simulink model "SistemaP1"  (R2023a)
settings: Solver=VariableStepAuto  StartTime=0.0  StopTime=10  RelTol=1e-3
libraries: slpidlib x1, simulink x1
settings Model: LastModifiedBy=biom3
settings DataIOCC: SaveOutput=off  ReturnWorkspaceOutputs=off  TimeSaveName=t
settings DebuggingCC: AlgebraicLoopMsg=none  ArtificialAlgebraicLoopMsg=none  InheritedTsInSrcMsg=none  MultiTaskCondExecSysMsg=none  TasksWithSamePriorityMsg=none  SigSpecEnsureSampleTimeMsg=none  UnknownTsInhSupMsg=none
settings RTWCC: GPUComputeCapability=5.0

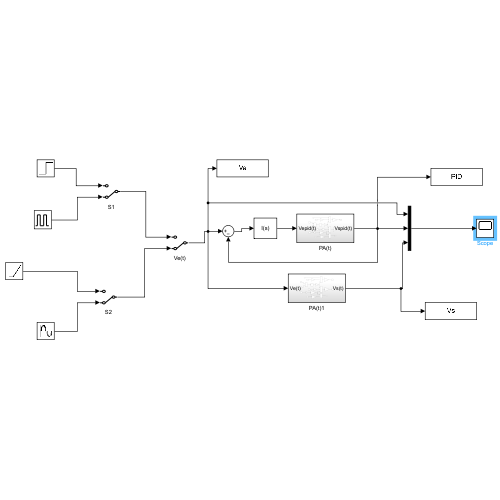
[thumbnail: Simulink's stored preview of the top-level diagram]
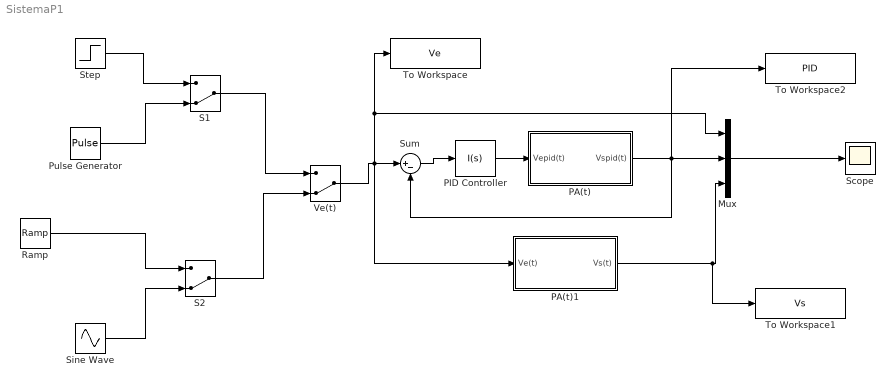
== system SistemaP1 ==
  Mux : Mux  Inputs=3
  PA(t) : Subsystem
  PA(t)1 : Subsystem
  PID Controller : slpidlib/PID Controller  Controller=I  Form=Parallel  TimeDomain=Continuous-time  UseExternalTs=off  SampleTime=-1  IntegratorMethod=Forward Euler  FilterMethod=Forward Euler  ControllerParametersSource=internal  P=1  I=731.453807138668  UseKiTs=off  D=1  N=1  UseFilter=on  TunerSelectOption=Transfer Function Based (PID Tuner App)  InitialConditionSource=internal  InitialConditionForIntegrator=0  InitialConditionForFilter=0  DifferentiatorICPrevScaledInput=0  ExternalReset=none  TrackingMode=off  Kt=1  LimitOutput=off  SatLimitsSource=internal  UpperSaturationLimit=inf  LowerSaturationLimit=-inf  LinearizeAsGain=on  AntiWindupMode=none  Kb=1  LimitIntegrator=off  UpperIntegratorSaturationLimit=inf  LowerIntegratorSaturationLimit=-inf  POutMin=[]  POutMax=[]  IOutMin=[]  IOutMax=[]  DOutMin=[]  DOutMax=[]  NOutMin=[]  NOutMax=[]  SumOutMin=[]  SumOutMax=[]  SaturationOutMin=[]  SaturationOutMax=[]  PParamMin=[]  PParamMax=[]  IParamMin=[]  IParamMax=[]  DParamMin=[]  DParamMax=[]  NParamMin=[]  NParamMax=[]  KbParamMin=[]  KbParamMax=[]  KtParamMin=[]  KtParamMax=[]  KbOutMin=[]  KbOutMax=[]  KtOutMin=[]  KtOutMax=[]  IntegratorOutMin=[]  IntegratorOutMax=[]  FilterOutMin=[]  FilterOutMax=[]  SumI1OutMin=[]  SumI1OutMax=[]  SumI2OutMin=[]  SumI2OutMax=[]  SumI3OutMin=[]  SumI3OutMax=[]  SumI4OutMin=[]  SumI4OutMax=[]  SumDOutMin=[]  SumDOutMax=[]  DifferentiatorOutMin=[]  DifferentiatorOutMax=[]  FilterDiffOutCoefMin=[]  FilterDiffOutCoefMax=[]  ReciprocalOutMin=[]  ReciprocalOutMax=[]  SumDenOutMin=[]  SumDenOutMax=[]  SumNumOutMin=[]  SumNumOutMax=[]  DivideOutMin=[]  DivideOutMax=[]  UdiffTsProdOutMin=[]  UdiffTsProdOutMax=[]  NTsProdOutMin=[]  NTsProdOutMax=[]  UintegralTsProdOutMin=[]  UintegralTsProdOutMax=[]  UngainTsProdOutMin=[]  UngainTsProdOutMax=[]  ClampingZeroOutDataTypeStr=Inherit: Inherit via back propagation  ClampingZeroOutMin=[]  ClampingZeroOutMax=[]  FilterDenConstantOutDataTypeStr=Inherit: Inherit via back propagation  FilterDenConstantOutMin=[]  FilterDenConstantOutMax=[]  PCopyOutDataTypeStr=Inherit: Inherit via back propagation  PCopyOutMin=[]  PCopyOutMax=[]  NCopyOutDataTypeStr=Inherit: Inherit via back propagation  NCopyOutMin=[]  NCopyOutMax=[]  IntegratorContinuousStateAttributes=''  IntegratorStateMustResolveToSignalObject=off  IntegratorRTWStateStorageClass=Auto  FilterContinuousStateAttributes=''  FilterStateMustResolveToSignalObject=off  FilterRTWStateStorageClass=Auto  ParallelPVariant=Disabled  IdealPVariant=Disabled  IVariant=InternalParameters  DVariant=Disabled  IntegratorVariant=Continuous  SatVariant=Disabled  AWVariant=Passthrough  PCopyVariant=Disabled  TRVariant=Disabled  FdbkBlocksVariant=Forward  IdealPFdbkVariant=Disabled  SatFdbkVariant=Disabled  DerivativeFilterVariant=Disabled  NVariant=Disabled  NCopyVariant=Disabled_SignalSpec  FilterICVariant=Disabled  IntegratorICVariant=InternalICs  ExternalResetVariant=Disabled  TRSumVariant=Passthrough  SumFdbkVariant=Disabled  SumVariant=Passthrough_I  TsampFilterVariant=InternalTs  TsampNgainVariant=Passthrough  TsampIntegralVariant=Disabled_SignalSpec  ExternalSaturationOutDataTypeStr=Inherit: Same as second input
  Pulse Generator : DiscretePulseGenerator  PulseType=Time based  Period=10  PulseWidth=10  PhaseDelay=1
  Ramp : simulink/Sources/Ramp  slope=1/10  start=0  InitialOutput=0
  S1 : ManualSwitch  CurrentSetting=0
  S2 : ManualSwitch  CurrentSetting=0
  Scope : Scope
  Sine Wave : Sin  Frequency=1.5708  SampleTime=0.001
  Step : Step  Time=0  SampleTime=0.001
  Sum : Sum  Inputs=|+-
  To Workspace : ToWorkspace  VariableName=Ve  SampleTime=-1
  To Workspace1 : ToWorkspace  VariableName=Vs  SampleTime=-1
  To Workspace2 : ToWorkspace  VariableName=PID  SampleTime=-1
  Ve(t) : ManualSwitch  CurrentSetting=0
  wires:
  Ramp/1 -> S2/1
  S1/1 -> Ve(t)/1
  Sine Wave/1 -> S2/2
  S2/1 -> Ve(t)/2
  Pulse Generator/1 -> S1/2
  Step/1 -> S1/1
  Mux/1 -> Scope/1
  Ve(t)/1 -> PA(t)1/1(Ve(t)), To Workspace/1, Mux/1, Sum/1
  Sum/1 -> PID Controller/1
  PA(t)1/1(Vs(t)) -> To Workspace1/1, Mux/3
  PA(t)/1(Vspid(t)) -> Sum/2, To Workspace2/1, Mux/2
  PID Controller/1 -> PA(t)/1(Vepid(t))

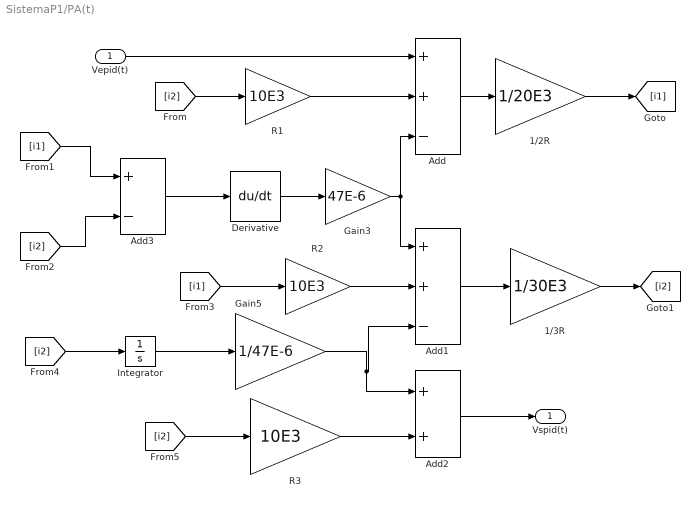
== system SistemaP1/PA(t) ==
  Vepid(t) : Inport
  1/2R : Gain  Gain=1/20E3
  1/3R : Gain  Gain=1/30E3
  Add : Sum  Inputs=++-
  Add1 : Sum  Inputs=++-
  Add2 : Sum
  Add3 : Sum  Inputs=+-
  Derivative : Derivative
  Gain3 : Gain  Gain=47E-6
  Gain5 : Gain  Gain=1/47E-6
  Integrator : Integrator
  R1 : Gain  Gain=10E3
  R2 : Gain  Gain=10E3
  R3 : Gain  Gain=10E3
  Vspid(t) : Outport
  wires:
  [i2] -> Integrator/1
  Add/1 -> 1/2R/1
  1/2R/1 -> [i1]
  [i2] -> Add3/2
  R3/1 -> Add2/2
  [i1] -> Add3/1
  Add3/1 -> Derivative/1
  1/3R/1 -> [i2]
  R1/1 -> Add/2
  Gain3/1 -> Add/3, Add1/1
  Integrator/1 -> Gain5/1
  [i1] -> R2/1
  [i2] -> R1/1
  R2/1 -> Add1/2
  Derivative/1 -> Gain3/1
  [i2] -> R3/1
  Add1/1 -> 1/3R/1
  Vepid(t)/1 -> Add/1
  Add2/1 -> Vspid(t)/1
  Gain5/1 -> Add2/1, Add1/3

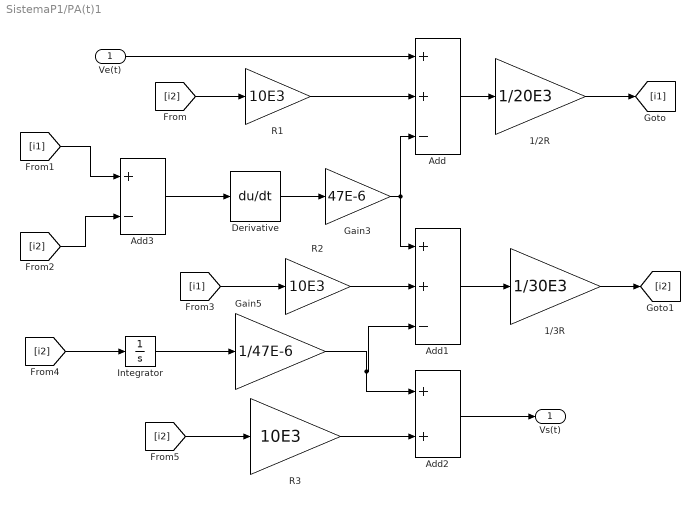
== system SistemaP1/PA(t)1 ==
  Ve(t) : Inport
  1/2R : Gain  Gain=1/20E3
  1/3R : Gain  Gain=1/30E3
  Add : Sum  Inputs=++-
  Add1 : Sum  Inputs=++-
  Add2 : Sum
  Add3 : Sum  Inputs=+-
  Derivative : Derivative
  Gain3 : Gain  Gain=47E-6
  Gain5 : Gain  Gain=1/47E-6
  Integrator : Integrator
  R1 : Gain  Gain=10E3
  R2 : Gain  Gain=10E3
  R3 : Gain  Gain=10E3
  Vs(t) : Outport
  wires:
  Ve(t)/1 -> Add/1
  Add2/1 -> Vs(t)/1
  [i2] -> R1/1
  R1/1 -> Add/2
  [i2] -> Add3/2
  [i1] -> Add3/1
  [i1] -> R2/1
  R2/1 -> Add1/2
  Add3/1 -> Derivative/1
  Derivative/1 -> Gain3/1
  Gain3/1 -> Add/3, Add1/1
  Add/1 -> 1/2R/1
  1/2R/1 -> [i1]
  Add1/1 -> 1/3R/1
  1/3R/1 -> [i2]
  Gain5/1 -> Add2/1, Add1/3
  Integrator/1 -> Gain5/1
  [i2] -> Integrator/1
  R3/1 -> Add2/2
  [i2] -> R3/1
